simulink model "cccv_charging"  (R2024b)
settings: Solver=ode23  StartTime=0.0  StopTime=1500  RelTol=1e-15
undefined symbols (not defined in the file): Ion, Lithium
libraries: spsMosfetLib x2, spsBatteryLib x1, spsControlledCurrentSourceLib x1, spsDCVoltageSourceLib x1, spsDiodeLib x1, spsSeriesRLCBranchLib x1, sps_lib x1
settings Model: Creator=vasudha  LastModifiedBy=vasudha
settings SolverCC: ZeroCrossControl=DisableAll
settings DebuggingCC: MaxConsecutiveZCsMsg=warning

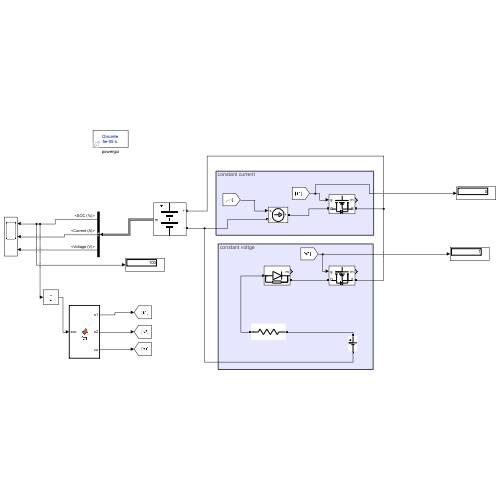
[thumbnail: Simulink's stored preview of the top-level diagram]
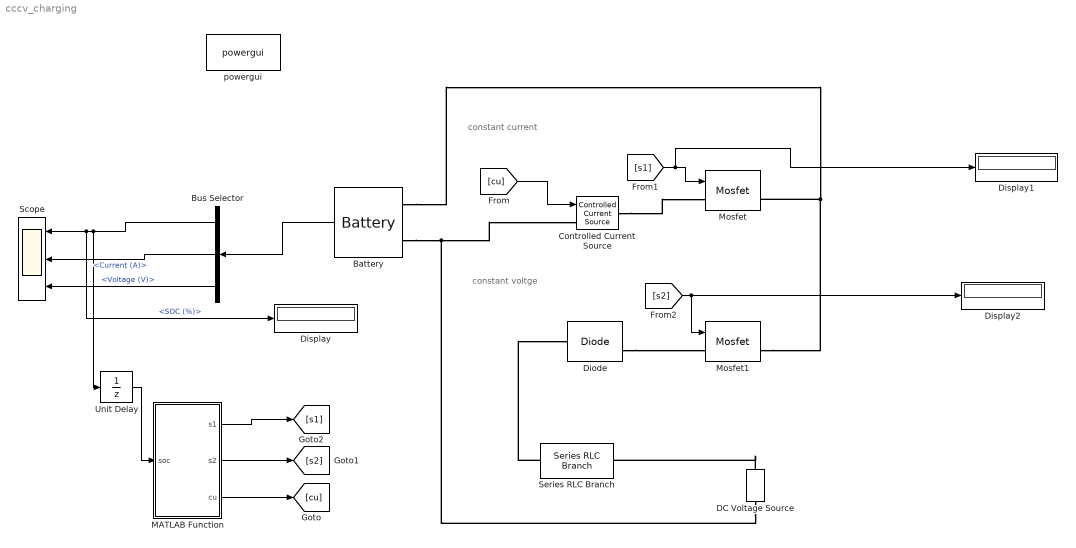
== system cccv_charging ==
  note: constant voltge
  note: constant current
  Battery : spsBatteryLib/Battery  BatType=Lithium-Ion  NomV=3.3  NomQ=2.3  SOC=79  Batt_Tr=30  PresetModel=on  MaxQ=2.3  MinV=2.475  FullV=3.8412  Dis_rate=1  R=0.014348  Normal_OP=2.08  expZone="[3.5653       0.113]"
  Bus Selector : BusSelector  OutputSignals=SOC (%),Current (A),Voltage (V)
  Controlled Current Source : spsControlledCurrentSourceLib/Controlled Current Source  Initialize=on  Source_Type=AC  Amplitude=0  Phase=0  Frequency=0  Measurements=None
  DC Voltage Source : spsDCVoltageSourceLib/DC Voltage Source  Amplitude=25  Measurements=None
  Diode : spsDiodeLib/Diode  Ron=0.001  Lon=0  Vf=0.8  IC=0  UseSnubber=0  Rs=500  Cs=250e-9  Measurements=on
  Display : Display
  Display1 : Display
  Display2 : Display
  MATLAB Function : MATLAB Function  TreatAsAtomicUnit=on
  Mosfet : spsMosfetLib/Mosfet  Ron=0.1  Lon=0  Rd=0.01  Vfd=0  IC=0  Rs=1e5  Cs=inf  Measurements=on
  Mosfet1 : spsMosfetLib/Mosfet  Ron=0.1  Lon=0  Rd=0.01  Vfd=0  IC=0  Rs=1e5  Cs=inf  Measurements=on
  Scope : Scope  NumInputPorts=3
  Series RLC Branch : spsSeriesRLCBranchLib/Series RLC Branch  LConnTagsString=__new0  RConnTagsString=__new0  BranchType=R  Resistance=1  Inductance=1e-3  SetiL0=off  InitialCurrent=0  Capacitance=1e-6  Setx0=off  InitialVoltage=0  Measurements=None
  Unit Delay : UnitDelay  SampleTime=-1  HasFrameUpgradeWarning=on
  powergui : sps_lib/powergui  Priority=1  SimulationMode=Discrete  SampleTime=5e-5  frequency=60  Iterations=50  frequencyindice=0  Pbase=100e6  ErrMax=1e-4  UnitsV=kV  UnitsW=MW  buscounter=0  FunctionMessages=off  echomessages=off  EnableUseOfTLC=off  CurrentSourceSwitches=off  DisableSnubberDevices=off  DisableRonSwitches=off  DisableVfSwitches=off  DisplayEquations=off  AutomaticDiscreteSolvers=off  SolverType=Tustin/Backward Euler (TBE)  Interpol=off  ExternalGateDelay=off  methode=off  Ts=100  x0status=blocks  SPID=on  SwTol=0  HookPort=off  NonlinearTolerance=1e-4  nMaxIteration=100  ContinueOnMaxIteration=off  RestoreLinks=warning  ResistiveCurrentMeasurement=off  Frange=[0:2:500]  Ylog=off  Xlog=on  ShowGrid=off  save=off  variable=ZData  structure=0  ZoomFFT=off  StartTime=0.0  cycles=1  DisplayStyle=1  fundamental=60  FreqAxis=off  MaxFrequency=1000  frequencyindicesteady=1  RmsSteady=1  display=off
  wires:
  Battery/1 -> Bus Selector/1
  Bus Selector/1 -> Unit Delay/1, Display/1, Scope/1  "<SOC (%)>"
  Bus Selector/2 -> Scope/2  "<Current (A)>"
  Bus Selector/3 -> Scope/3  "<Voltage (V)>"
  MATLAB Function/3(cu) -> [cu]
  [cu] -> Controlled Current Source/1
  MATLAB Function/2(s2) -> [s2]
  MATLAB Function/1(s1) -> [s1]
  [s1] -> Display1/1, Mosfet/1
  [s2] -> Mosfet1/1, Display2/1
  Unit Delay/1 -> MATLAB Function/1(soc)
  connections:
  Battery/LConn2 -- Controlled Current Source/LConn1 -- DC Voltage Source/LConn1
  Controlled Current Source/RConn1 -- Mosfet/LConn1
  Battery/LConn1 -- Mosfet1/RConn1 -- Mosfet/RConn1
  Diode/RConn1 -- Mosfet1/LConn1
  DC Voltage Source/RConn1 -- Series RLC Branch/RConn1
  Series RLC Branch/LConn1 -- Diode/LConn1

== matlab function cccv_charging/MATLAB Function ==
  data: soc input; s1 output; s2 output; cu output
function [s1, s2, cu] = fcn(soc)
cu = 0; % Initialize cu
s1 = 0; % Initialize s1
s2 = 0; % Initialize s2

if (soc == 0) || (soc <= 80)
    s1 = 1;
    s2 = 0;
    cu = 2;
else
    s1 = 0;
    s2 = 1;
end
